simulink model "TwoLinkCartesian"  (Simulink 7.6)
settings: Solver=ode45  StartTime=0.0  StopTime=10.0  RelTol=1e-3
libraries: roblocks x3, simulink x1
settings Model: Creator=mahyar  LastModifiedBy=mahyar

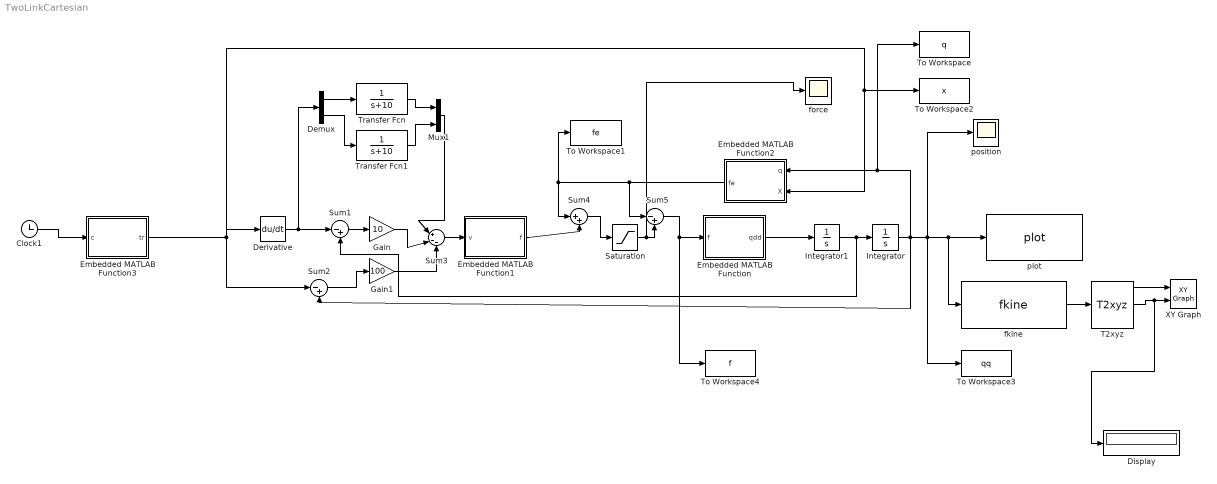
== system TwoLinkCartesian ==
  Clock1 : Clock
      settings: Decimation=10
  Demux : Demux  Outputs=2
  Derivative : Derivative
  Display : Display
  Embedded MATLAB Function : Stateflow chart  TreatAsAtomicUnit=on
  Embedded MATLAB Function1 : Stateflow chart  TreatAsAtomicUnit=on
  Embedded MATLAB Function2 : Stateflow chart  TreatAsAtomicUnit=on
  Embedded MATLAB Function3 : Stateflow chart  TreatAsAtomicUnit=on
  Gain : Gain  Gain=10
  Gain1 : Gain  Gain=100
  Integrator : Integrator  InitialCondition=[0;0]
  Integrator1 : Integrator  InitialCondition=[0 ;0]
  Mux1 : Mux  Inputs=2
  Saturation : Saturate  UpperLimit=80  LowerLimit=-80
  Sum1 : Sum  Inputs=|-+
  Sum2 : Sum  Inputs=|-+
  Sum3 : Sum  Inputs=|+--
  Sum4 : Sum  Inputs=|++
  Sum5 : Sum  Inputs=|-+
  T2xyz : roblocks/T2xyz  SystemSampleTime=-1
  To Workspace : ToWorkspace  VariableName=q  SampleTime=-1  SaveFormat=Structure
  To Workspace1 : ToWorkspace  VariableName=fe  SampleTime=-1  SaveFormat=Structure
  To Workspace2 : ToWorkspace  VariableName=x  SampleTime=-1  SaveFormat=Structure
  To Workspace3 : ToWorkspace  VariableName=qq  SampleTime=-1  SaveFormat=Structure
  To Workspace4 : ToWorkspace  VariableName=f  SampleTime=-1  SaveFormat=Structure
  Transfer Fcn : TransferFcn  Denominator=[1 10]
  Transfer Fcn1 : TransferFcn  Denominator=[1 10]
  XY Graph : simulink/Sinks/XY Graph  SystemSampleTime=-1  xmin=-4  xmax=4  ymin=-4  ymax=4  st=-1
  fkine : roblocks/fkine  SystemSampleTime=-1  robot=r
  force : Scope
      settings: TimeRange=10  YMin=-20  YMax=80  SaveName=ScopeData2
  plot : roblocks/plot  SystemSampleTime=-1  robot=r
  position : Scope
      settings: YMin=0  YMax=1.2
  wires:
  fkine/1 -> T2xyz/1
  Embedded MATLAB Function/1(qdd) -> Integrator1/1
  Integrator/1 -> plot/1, fkine/1, position/1, To Workspace3/1, Sum2/2, Embedded MATLAB Function2/1(q), To Workspace/1
  Integrator1/1 -> Integrator/1, Sum1/2
  Derivative/1 -> Sum1/1, Demux/1
  Sum3/1 -> Embedded MATLAB Function1/1(v)
  Sum1/1 -> Gain/1
  Gain/1 -> Sum3/2
  Sum2/1 -> Gain1/1
  Gain1/1 -> Sum3/3
  Demux/1 -> Transfer Fcn/1
  Demux/2 -> Transfer Fcn1/1
  Transfer Fcn/1 -> Mux1/1
  Transfer Fcn1/1 -> Mux1/2
  Mux1/1 -> Sum3/1
  Embedded MATLAB Function2/1(fe) -> Sum5/1, Sum4/1, To Workspace1/1
  Embedded MATLAB Function1/1(f) -> Sum4/2
  Embedded MATLAB Function3/1(tr) -> Derivative/1, Sum2/1, Embedded MATLAB Function2/2(X), To Workspace2/1
  T2xyz/1 -> XY Graph/1
  T2xyz/2 -> XY Graph/2, Display/1
  Sum5/1 -> Embedded MATLAB Function/1(f), To Workspace4/1
  Sum4/1 -> Saturation/1
  Saturation/1 -> Sum5/2, force/1
  Clock1/1 -> Embedded MATLAB Function3/1(c)

== matlab function Embedded MATLAB Function2 ==
  data: q input double; fe output double; X input double
function fe = fcn(q,X)
k = 150000;
z = q(1);
x = q(2);
if  (z>.5 && z<.6) || x<.5
    fe = [0;0];
else
     fe1 = 0;
     fe2 = k*(x-X(2));
     fe = [fe1;fe2];
end

== matlab function Embedded MATLAB Function3 ==
  data: tr output double; c input double
function tr = fcn(c)

% if c < 8
% tr = [.55 ; 0];
% else
%     tr = [.55 ; 1];
% end
% 
tr = [.6;.6];

== matlab function Embedded MATLAB Function ==
  data: f input double; qdd output double
function qdd= fcn(f)
m1 = 1;
m2 = 1;
g = 9.8;
M = [m1+m2 , 0; 0,m2];
G = [g*(m1+m2);0];
qdd = inv(M)*(f-G) ;

== matlab function Embedded MATLAB Function1 ==
  data: v input double; f output double
function f = fcn(v)

m1 = 1;
m2 = 1;
g = 9.8;
M = [m1+m2 , 0; 0,m2];
G = [g*(m1+m2);0];
f = G+M*v;
